simulink model "untitled"  (R2021a)
settings: Solver=VariableStepAuto  StartTime=0.0  StopTime=100  RelTol=1e-3
settings Model: Creator=fedor  LastModifiedBy=fedor

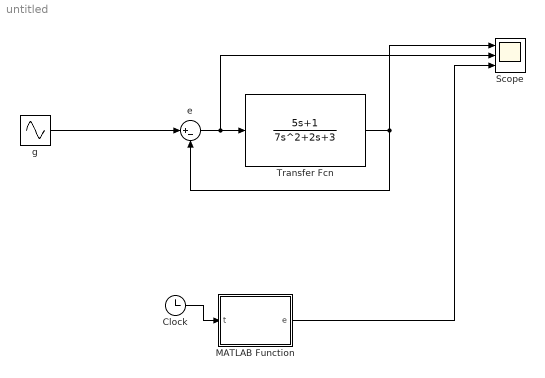
== system untitled ==
  Clock : Clock
  MATLAB Function : MATLAB Function  TreatAsAtomicUnit=on
  Scope : Scope  NumInputPorts=3
  Transfer Fcn : TransferFcn  Numerator=[5 1]  Denominator=[7 2 3]
  e : Sum  Inputs=|+-
  g : Sin  Amplitude=8  Frequency=2  Phase=1  SampleTime=0
  wires:
  e/1 -> Scope/2, Transfer Fcn/1
  Transfer Fcn/1 -> e/2, Scope/1
  g/1 -> e/1
  Clock/1 -> MATLAB Function/1(t)
  MATLAB Function/1(e) -> Scope/3

== matlab function untitled/MATLAB Function ==
  data: t input; e output
function e = fcn(t)
s = 1i*2;
W = (5*s+1)/(7*s^2+2*s+3);
W_1 = 1/(1+W);
A=abs(W_1);
f= angle(W_1);
e = 8*A*sin(2*t+1+f);
